simulink model "test"  (R2022a)
settings: Solver=VariableStepAuto  StartTime=0.0  StopTime=10.0  RelTol=1e-3
undefined symbols (not defined in the file or in its folder): phi, r, sigbuilder_block, theta
libraries: robotgazebolib x5
settings Model: Creator=abiyyumufti  LastModifiedBy=abiyyumufti

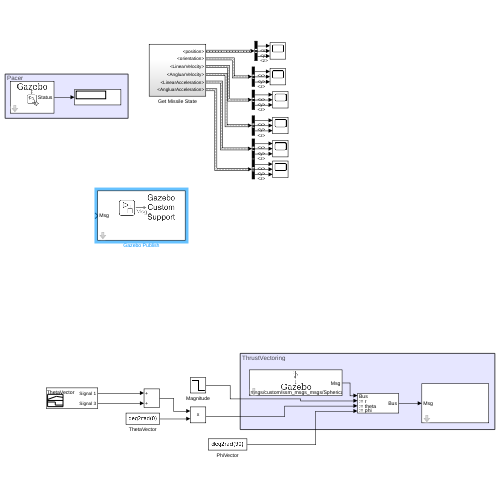
[thumbnail: Simulink's stored preview of the top-level diagram]
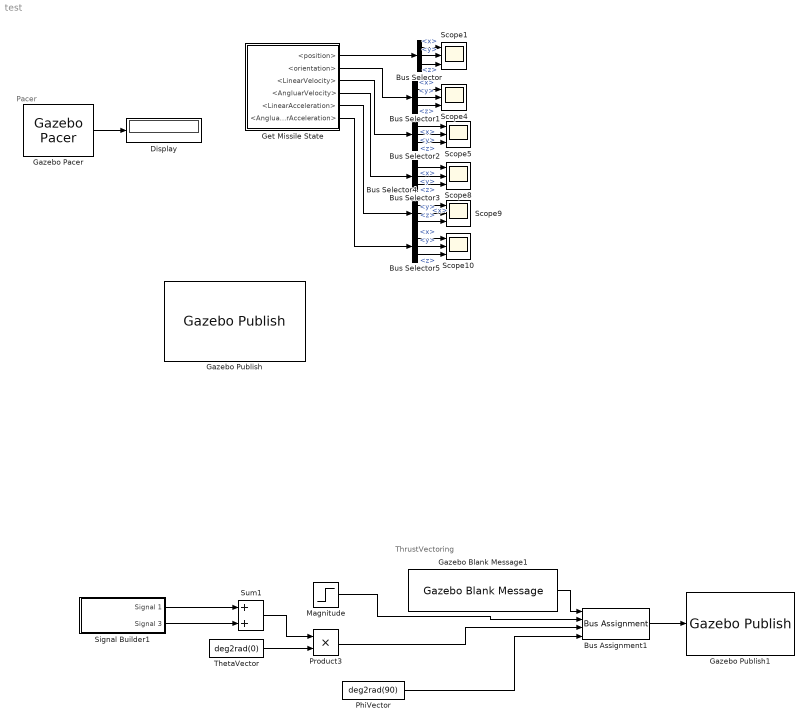
== system test ==
  note: Pacer
  note: ThrustVectoring
  Bus Assignment1 : BusAssignment  AssignedSignals=r,theta,phi
  Bus Selector{,1..5} (6 alike) : BusSelector  OutputSignals=x,y,z
  Display : Display
  Gazebo Blank Message1 : robotgazebolib/Gazebo Blank Message  msgType=gazebo_msgs/custom/ssm_msgs_msgs/SphericalVector  sampleTime=0.001  busName='Gazebo_SL_Bus_gazebo_msgs_custom_ssm_msgs_msgs_SphericalVector'
      settings: SourceProductBaseCode=RO
  Gazebo Pacer : robotgazebolib/Gazebo Pacer  ResetBehavior=Reset Gazebo simulation time and scene  SampleTime=0.001
      settings: SourceProductBaseCode=RO
  Gazebo Publish : robotgazebolib/Gazebo Publish  topicSource=From Gazebo  topic=/my_topic  messageType=gazebo_msgs/TestPose  sampleTime=0.001
      settings: SourceProductBaseCode=RO
  Gazebo Publish1 : robotgazebolib/Gazebo Publish  topicSource=Specify your own  topic=/gazebo/my_world/thrust_force  messageType=gazebo_msgs/custom/ssm_msgs_msgs/SphericalVector  sampleTime=0.001
      settings: SourceProductBaseCode=RO
  Get Missile State : Subsystem
  Magnitude : Step  Time=2  Before=80000  After=16000  SampleTime=0
  PhiVector : Constant  Value=deg2rad(90)
  Product3 : Product
  Scope{1,4..5,8..10} (6 alike) : Scope  NumInputPorts=3
  Signal Builder1 : Subsystem  Tag=STV Subsys  LoadFcn=sigbuilder_block('load');  StartFcn=sigbuilder_block('start');  StopFcn=sigbuilder_block('stop');  ClipboardFcn=sigbuilder_block('clipboard');  mask(Sigbuilder block){tuvar=[0:10]}
      mask help: Simulink:masks:SigbuilderBlock_MD
      mask init:
      | if ~strcmp(get_param(bdroot(gcbh),'SimulationStatus'),'stopped') tuvar = sigbuilder_block('maskInit'); end
      settings: CopyFcn=sigbuilder_block('copy');  DeleteFcn=sigbuilder_block('delete');  ModelCloseFcn=sigbuilder_block('modelClose');  PreSaveFcn=sigbuilder_block('preSave');  PauseFcn=sigbuilder_block('pause');  ContinueFcn=sigbuilder_block('continue');  NameChangeFcn=sigbuilder_block('namechange');  OpenFcn=sigbuilder_block('open',[40.5 0 1399.5 658.5 ]);  CloseFcn=sigbuilder_block('close');
      mask Display: plot(0, 0, 100, 100,[2, 2, 32, 32, 2], [68, 8, 8, 68, 68],[32, 2], [38, 38], [32, 19, 2],[53, 60, 44], [32, 17, 17, 2],[16, 16, 31, 31]);txt = getActiveGroup(gcbh);text(2, 100, txt,'verticalAlignment', 'top');
  Sum1 : Sum
  ThetaVector : Constant  Value=deg2rad(0)
  wires:
  Gazebo Pacer/1 -> Display/1
  Get Missile State/5(<LinearAcceleration>) -> Bus Selector4/1
  Bus Selector2/3 -> Scope5/3  "<z>"
  Bus Selector4/2 -> Scope9/2  "<y>"
  Bus Selector3/1 -> Scope8/1  "<x>"
  Get Missile State/6(<AngluarAcceleration>) -> Bus Selector5/1
  Bus Selector2/1 -> Scope5/1  "<x>"
  Bus Selector1/2 -> Scope4/2  "<y>"
  Bus Selector3/3 -> Scope8/3  "<z>"
  Bus Selector/3 -> Scope1/3  "<z>"
  Bus Selector5/2 -> Scope10/2  "<y>"
  Bus Selector2/2 -> Scope5/2  "<y>"
  Bus Selector5/3 -> Scope10/3  "<z>"
  Bus Selector/2 -> Scope1/2  "<y>"
  Get Missile State/1(<position>) -> Bus Selector/1
  Bus Selector4/1 -> Scope9/1  "<x>"
  Bus Selector5/1 -> Scope10/1  "<x>"
  Get Missile State/2(<orientation>) -> Bus Selector1/1
  Bus Selector1/1 -> Scope4/1  "<x>"
  Bus Selector3/2 -> Scope8/2  "<y>"
  Get Missile State/3(<LinearVelocity>) -> Bus Selector2/1
  Bus Selector1/3 -> Scope4/3  "<z>"
  Get Missile State/4(<AngluarVelocity>) -> Bus Selector3/1
  Bus Selector4/3 -> Scope9/3  "<z>"
  Bus Selector/1 -> Scope1/1  "<x>"
  PhiVector/1 -> Bus Assignment1/4
  Signal Builder1/1(Signal 1) -> Sum1/1
  Gazebo Blank Message1/1 -> Bus Assignment1/1
  Sum1/1 -> Product3/1
  Product3/1 -> Bus Assignment1/3
  Signal Builder1/2(Signal 3) -> Sum1/2
  Bus Assignment1/1 -> Gazebo Publish1/1
  ThetaVector/1 -> Product3/2
  Magnitude/1 -> Bus Assignment1/2

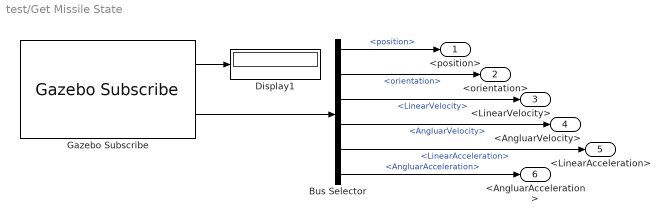
== system test/Get Missile State ==
  Bus Selector : BusSelector  OutputSignals=Pose.position,Pose.orientation,LinearVelocity,AngluarVelocity,LinearAcceleration,AngluarAcceleration
  Display1 : Display
  Gazebo Subscribe : robotgazebolib/Gazebo Subscribe  topicSource=From Gazebo  topic=/gazebo/my_world/DynamicState  messageType=gazebo_msgs/custom/ssm_msgs_msgs/DynamicState  sampleTime=0.001
      settings: SourceProductBaseCode=RO
  <position> : Outport
  <orientation> : Outport  Port=2
  <LinearVelocity> : Outport  Port=3
  <AngluarVelocity> : Outport  Port=4
  <LinearAcceleration> : Outport  Port=5
  <AngluarAcceleration> : Outport  Port=6
  wires:
  Gazebo Subscribe/2 -> Bus Selector/1
  Gazebo Subscribe/1 -> Display1/1
  Bus Selector/4 -> <AngluarVelocity>/1  "<AngluarVelocity>"
  Bus Selector/6 -> <AngluarAcceleration>/1  "<AngluarAcceleration>"
  Bus Selector/5 -> <LinearAcceleration>/1  "<LinearAcceleration>"
  Bus Selector/1 -> <position>/1  "<position>"
  Bus Selector/3 -> <LinearVelocity>/1  "<LinearVelocity>"
  Bus Selector/2 -> <orientation>/1  "<orientation>"

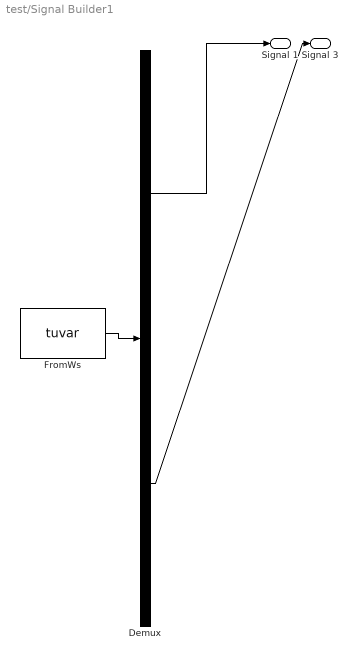
== system test/Signal Builder1 ==
  Demux : Demux  Tag=STV Demux  Outputs=2
      settings: DisplayOption=none
  FromWs : FromWorkspace  Tag=STV FromWs  VariableName=tuvar
      SigBuilderData=|
      | common.afterFinalStr = 'Extrapolate'
      | common.sampleTime = 0
      | dataSet.timeRange = [0 60]
      | dataSet.name = 'ThetaVector'
      | sbobj.Groups.Name = 'ThetaVector'
      | sbobj.Groups.Signals(1).Name = 'Signal 1'
      | sbobj.Groups.Signals(1).XData = [0 1 2 3 60]
      | sbobj.Groups.Signals(1).YData = [0 0 1 0 0]
      | sbobj.Groups.Signals(2).Name = 'Signal 3'
      | sbobj.Groups.Signals(2).XData = [0 3 4 5 60]
      | sbobj.Groups.Signals(2).YData = [0 0 -2 0 0]
      | sbobj.Groups.TimeRange = [0 60]
  Signal 1 : Outport  Tag=STV Outport
  Signal 3 : Outport  Tag=STV Outport  Port=2
  wires:
  FromWs/1 -> Demux/1
  Demux/1 -> Signal 1/1
  Demux/2 -> Signal 3/1
